simulink model "Model_120S2P"  (R2019b)
settings: Solver=VariableStepAuto  StartTime=0.0  StopTime=800  RelTol=1e-3
libraries: fl_lib x29, nesl_utility x6, simulink x2, hwlogiciolib x1, ee_lib x1
(part 2 of 3)

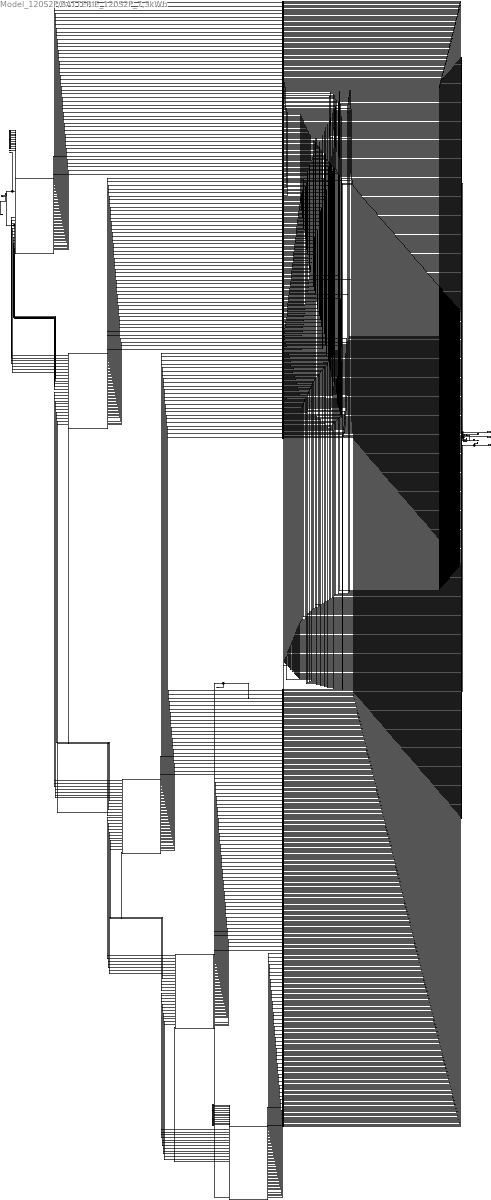
== system Model_120S2P/BATTERIE_120S2P_7,3kWh ==
  Bus Creator : BusCreator  Inputs=240
  Bus Creator1 : BusCreator  Inputs=240
  Bus Creator2 : BusCreator  Inputs=240
  Bus Selector{,1..239} (240 alike) : BusSelector  OutputSignals=Temperature,SOC,Voltage
  Compare To Constant1 : simulink/Logic and Bit Operations/Compare To Constant  relop=<=  const=0.05  OutDataTypeStr=boolean
  Compare To Constant2 : simulink/Logic and Bit Operations/Compare To Constant  relop=>  const=60.5  OutDataTypeStr=boolean
  Electrical Reference : fl_lib/Electrical/Electrical Elements/Electrical Reference
  MinMax1 : MinMax
  MinMax2 : MinMax  Function=max
  OCV : Scope
  OR : Logic  Operator=OR  IconShape=distinctive  AllPortsSameDT=off  OutDataTypeStr=boolean
  PS-Simulink Converter : nesl_utility/PS-Simulink Converter  PhysicalDomain=network_engine_domain  SubClassName=ps_output  LeftPortType=input  RightPortType=output  PseudoPeriodic=off  Frequencies=[]  Unit=inherit  AffineConversion=off
  Scope : Scope
  Subsystem{,1..4} (5 alike) : Subsystem  ReferencedSubsystem=segment_24S2P
  Temperature Source{1..24} (24 alike) : fl_lib/Thermal/Thermal Sources/Temperature Source  temperature=cell_prop.T_ext K
      settings: SourceProductName=Simscape
  To Workspace : ToWorkspace  VariableName=temperature  SaveFormat=Timeseries  SampleTime=-1
  To Workspace1 : ToWorkspace  VariableName=voltage  SaveFormat=Timeseries  SampleTime=-1
  To Workspace2 : ToWorkspace  VariableName=soc  SaveFormat=Timeseries  SampleTime=-1
  Voltage Sensor : fl_lib/Electrical/Electrical Sensors/Voltage Sensor
  + : PMIOPort  Side=Left
  - : PMIOPort  Port=2  Side=Left
  LED : Outport
  TEMP : Outport  Port=2
  SOC : Outport  Port=3
  wires:
  Bus Selector197/2 -> Bus Creator2/210  "<SOC>"
  Bus Selector199/3 -> Bus Creator1/212  "<Voltage>"
  Bus Selector226/3 -> Bus Creator1/222  "<Voltage>"
  Bus Selector191/3 -> Bus Creator1/156  "<Voltage>"
  Bus Selector119/2 -> Bus Creator2/100  "<SOC>"
  Bus Selector161/2 -> Bus Creator2/181  "<SOC>"
  Bus Selector107/2 -> Bus Creator2/116  "<SOC>"
  Bus Selector139/1 -> Bus Creator/102  "<Temperature>"
  Bus Selector72/2 -> Bus Creator2/87  "<SOC>"
  Bus Selector156/3 -> Bus Creator1/168  "<Voltage>"
  Bus Selector173/3 -> Bus Creator1/190  "<Voltage>"
  Subsystem2/14 -> Bus Selector101/1
  Subsystem3/31 -> Bus Selector179/1
  Subsystem4/31 -> Bus Selector227/1
  Subsystem4/5 -> Bus Selector222/1
  Subsystem/41 -> Bus Selector32/1
  Bus Selector213/2 -> Bus Creator2/232  "<SOC>"
  Bus Selector160/2 -> Bus Creator2/180  "<SOC>"
  Subsystem/14 -> Bus Selector13/1
  Bus Selector128/1 -> Bus Creator/144  "<Temperature>"
  Subsystem/4 -> Bus Selector3/1
  Bus Selector52/3 -> Bus Creator1/61  "<Voltage>"
  Bus Selector42/1 -> Bus Creator/29  "<Temperature>"
  Bus Selector15/3 -> Bus Creator1/16  "<Voltage>"
  Bus Selector227/2 -> Bus Creator2/223  "<SOC>"
  Subsystem2/13 -> Bus Selector100/1
  Bus Selector136/2 -> Bus Creator2/128  "<SOC>"
  Bus Selector28/2 -> Bus Creator2/37  "<SOC>"
  Bus Selector15/2 -> Bus Creator2/16  "<SOC>"
  Bus Selector108/2 -> Bus Creator2/99  "<SOC>"
  Bus Selector36/1 -> Bus Creator/27  "<Temperature>"
  Subsystem/39 -> Bus Selector30/1
  Bus Selector183/3 -> Bus Creator1/150  "<Voltage>"
  Subsystem/23 -> Bus Selector22/1
  Subsystem/48 -> Bus Selector38/1
  Bus Selector105/2 -> Bus Creator2/114  "<SOC>"
  Bus Selector163/1 -> Bus Creator/148  "<Temperature>"
  Subsystem3/24 -> Bus Selector156/1
  Bus Selector195/3 -> Bus Creator1/208  "<Voltage>"
  Bus Selector55/1 -> Bus Creator/64  "<Temperature>"
  Bus Selector113/3 -> Bus Creator1/121  "<Voltage>"
  Bus Selector59/1 -> Bus Creator/68  "<Temperature>"
  Subsystem3/17 -> Bus Selector148/1
  Bus Selector70/3 -> Bus Creator1/86  "<Voltage>"
  Bus Selector73/1 -> Bus Creator/88  "<Temperature>"
  Bus Selector74/1 -> Bus Creator/89  "<Temperature>"
  Subsystem2/33 -> Bus Selector137/1
  Bus Selector231/1 -> Bus Creator/198  "<Temperature>"
  Bus Selector190/3 -> Bus Creator1/155  "<Voltage>"
  Bus Selector101/2 -> Bus Creator2/110  "<SOC>"
  Bus Selector37/1 -> Bus Creator/45  "<Temperature>"
  Bus Selector136/3 -> Bus Creator1/128  "<Voltage>"
  Bus Selector42/3 -> Bus Creator1/29  "<Voltage>"
  Subsystem2/9 -> Bus Selector142/1
  Subsystem2/42 -> Bus Selector123/1
  Bus Selector214/1 -> Bus Creator/233  "<Temperature>"
  Bus Selector238/1 -> Bus Creator/203  "<Temperature>"
  Bus Selector202/2 -> Bus Creator2/214  "<SOC>"
  Bus Selector57/1 -> Bus Creator/66  "<Temperature>"
  Bus Selector24/3 -> Bus Creator1/25  "<Voltage>"
  Bus Selector171/3 -> Bus Creator1/189  "<Voltage>"
  Bus Selector71/2 -> Bus Creator2/52  "<SOC>"
  Bus Selector206/3 -> Bus Creator1/218  "<Voltage>"
  Bus Selector55/3 -> Bus Creator1/64  "<Voltage>"
  Subsystem3/9 -> Bus Selector186/1
  Bus Selector170/2 -> Bus Creator2/171  "<SOC>"
  Bus Selector149/1 -> Bus Creator/162  "<Temperature>"
  Bus Selector176/2 -> Bus Creator2/172  "<SOC>"
  Subsystem3/1 -> Bus Selector188/1
  Bus Selector19/3 -> Bus Creator1/20  "<Voltage>"
  Bus Selector153/3 -> Bus Creator1/165  "<Voltage>"
  Bus Selector164/2 -> Bus Creator2/183  "<SOC>"
  Bus Selector153/2 -> Bus Creator2/165  "<SOC>"
  Bus Selector133/2 -> Bus Creator2/125  "<SOC>"
  Bus Selector47/2 -> Bus Creator2/34  "<SOC>"
  Bus Selector106/2 -> Bus Creator2/115  "<SOC>"
  Subsystem1/46 -> Bus Selector81/1
  Bus Selector213/3 -> Bus Creator1/232  "<Voltage>"
  Bus Selector30/1 -> Bus Creator/39  "<Temperature>"
  Bus Selector179/2 -> Bus Creator2/175  "<SOC>"
  Bus Selector150/1 -> Bus Creator/163  "<Temperature>"
  Bus Selector18/1 -> Bus Creator/19  "<Temperature>"
  Bus Selector68/3 -> Bus Creator1/84  "<Voltage>"
  Bus Selector111/1 -> Bus Creator/119  "<Temperature>"
  Bus Selector141/2 -> Bus Creator2/104  "<SOC>"
  Bus Selector45/2 -> Bus Creator2/32  "<SOC>"
  Subsystem1/28 -> Bus Selector84/1
  Bus Selector77/2 -> Bus Creator2/92  "<SOC>"
  Subsystem1/22 -> Bus Selector62/1
  Bus Selector34/3 -> Bus Creator1/43  "<Voltage>"
  Subsystem4/47 -> Bus Selector223/1
  Subsystem3/38 -> Bus Selector162/1
  Bus Selector157/2 -> Bus Creator2/169  "<SOC>"
  Bus Selector199/2 -> Bus Creator2/212  "<SOC>"
  Subsystem1/45 -> Bus Selector79/1
  Bus Selector39/2 -> Bus Creator2/46  "<SOC>"
  Bus Selector7/2 -> Bus Creator2/8  "<SOC>"
  Subsystem4/15 -> Bus Selector194/1
  Bus Selector161/3 -> Bus Creator1/181  "<Voltage>"
  Bus Selector119/3 -> Bus Creator1/100  "<Voltage>"
  Bus Selector182/1 -> Bus Creator/178  "<Temperature>"
  Bus Selector4/2 -> Bus Creator2/5  "<SOC>"
  Bus Selector75/2 -> Bus Creator2/90  "<SOC>"
  Bus Selector113/1 -> Bus Creator/121  "<Temperature>"
  Bus Selector57/2 -> Bus Creator2/66  "<SOC>"
  Bus Selector44/2 -> Bus Creator2/31  "<SOC>"
  Bus Selector109/2 -> Bus Creator2/117  "<SOC>"
  Bus Selector120/2 -> Bus Creator2/135  "<SOC>"
  Bus Selector137/3 -> Bus Creator1/129  "<Voltage>"
  Bus Selector143/2 -> Bus Creator2/106  "<SOC>"
  Subsystem4/28 -> Bus Selector224/1
  Subsystem/38 -> Bus Selector29/1
  Bus Selector235/3 -> Bus Creator1/202  "<Voltage>"
  Bus Selector218/2 -> Bus Creator2/219  "<SOC>"
  Bus Selector200/1 -> Bus Creator/195  "<Temperature>"
  Bus Selector165/1 -> Bus Creator/184  "<Temperature>"
  Bus Selector134/1 -> Bus Creator/126  "<Temperature>"
  Bus Selector117/3 -> Bus Creator1/133  "<Voltage>"
  Subsystem2/1 -> Bus Selector96/1
  Bus Selector102/3 -> Bus Creator1/111  "<Voltage>"
  Bus Selector134/3 -> Bus Creator1/126  "<Voltage>"
  Bus Selector217/3 -> Bus Creator1/236  "<Voltage>"
  Bus Selector223/3 -> Bus Creator1/239  "<Voltage>"
  Bus Selector130/3 -> Bus Creator1/101  "<Voltage>"
  Bus Selector227/3 -> Bus Creator1/223  "<Voltage>"
  Bus Selector31/3 -> Bus Creator1/40  "<Voltage>"
  Bus Selector212/3 -> Bus Creator1/231  "<Voltage>"
  Bus Selector222/1 -> Bus Creator/197  "<Temperature>"
  Bus Selector223/1 -> Bus Creator/239  "<Temperature>"
  Bus Selector43/1 -> Bus Creator/30  "<Temperature>"
  Bus Selector78/2 -> Bus Creator2/75  "<SOC>"
  Bus Selector191/2 -> Bus Creator2/156  "<SOC>"
  Bus Selector177/3 -> Bus Creator1/173  "<Voltage>"
  Subsystem/6 -> Bus Selector5/1
  Bus Selector112/2 -> Bus Creator2/120  "<SOC>"
  Bus Selector22/2 -> Bus Creator2/23  "<SOC>"
  Subsystem/10 -> Bus Selector9/1
  Subsystem2/5 -> Bus Selector130/1
  Bus Selector90/3 -> Bus Creator1/82  "<Voltage>"
  Bus Selector140/1 -> Bus Creator/103  "<Temperature>"
  Bus Selector89/1 -> Bus Creator/81  "<Temperature>"
  Bus Selector180/3 -> Bus Creator1/176  "<Voltage>"
  Bus Selector117/2 -> Bus Creator2/133  "<SOC>"
  Bus Selector180/2 -> Bus Creator2/176  "<SOC>"
  Bus Selector45/1 -> Bus Creator/32  "<Temperature>"
  Subsystem4/29 -> Bus Selector225/1
  Bus Selector225/3 -> Bus Creator1/221  "<Voltage>"
  Bus Selector225/2 -> Bus Creator2/221  "<SOC>"
  Bus Creator1/1 -> OCV/1, To Workspace1/1
  Bus Selector64/2 -> Bus Creator2/72  "<SOC>"
  Bus Selector116/2 -> Bus Creator2/132  "<SOC>"
  Bus Selector231/2 -> Bus Creator2/198  "<SOC>"
  Bus Creator2/1 -> MinMax1/1, SOC/1, To Workspace2/1
  Subsystem3/37 -> Bus Selector161/1
  Subsystem3/8 -> Bus Selector185/1
  Subsystem1/21 -> Bus Selector61/1
  Bus Selector189/1 -> Bus Creator/146  "<Temperature>"
  Bus Selector150/3 -> Bus Creator1/163  "<Voltage>"
  Subsystem/32 -> Bus Selector45/1
  Bus Creator/1 -> MinMax2/1, TEMP/1, To Workspace/1
  Subsystem1/31 -> Bus Selector87/1
  Bus Selector9/1 -> Bus Creator/10  "<Temperature>"
  Subsystem1/27 -> Bus Selector78/1
  Bus Selector22/1 -> Bus Creator/23  "<Temperature>"
  Bus Selector154/1 -> Bus Creator/166  "<Temperature>"
  Bus Selector11/2 -> Bus Creator2/12  "<SOC>"
  Subsystem1/39 -> Bus Selector72/1
  Bus Selector60/2 -> Bus Creator2/51  "<SOC>"
  Subsystem1/36 -> Bus Selector68/1
  Bus Selector80/2 -> Bus Creator2/96  "<SOC>"
  Bus Selector12/2 -> Bus Creator2/13  "<SOC>"
  Subsystem2/26 -> Bus Selector114/1
  Subsystem3/30 -> Bus Selector178/1
  Bus Selector171/2 -> Bus Creator2/189  "<SOC>"
  Bus Selector11/3 -> Bus Creator1/12  "<Voltage>"
  Bus Selector85/3 -> Bus Creator1/77  "<Voltage>"
  Bus Selector220/3 -> Bus Creator1/240  "<Voltage>"
  Bus Selector34/2 -> Bus Creator2/43  "<SOC>"
  Bus Selector233/1 -> Bus Creator/200  "<Temperature>"
  Bus Selector184/3 -> Bus Creator1/151  "<Voltage>"
  Bus Selector82/1 -> Bus Creator/53  "<Temperature>"
  Bus Selector228/2 -> Bus Creator2/224  "<SOC>"
  Bus Selector93/2 -> Bus Creator2/56  "<SOC>"
  Subsystem4/43 -> Bus Selector216/1
  Subsystem2/15 -> Bus Selector102/1
  Bus Selector64/3 -> Bus Creator1/72  "<Voltage>"
  Bus Selector43/3 -> Bus Creator1/30  "<Voltage>"
  Bus Selector152/3 -> Bus Creator1/147  "<Voltage>"
  Subsystem4/21 -> Bus Selector201/1
  Subsystem4/27 -> Bus Selector218/1
  Bus Selector221/2 -> Bus Creator2/238  "<SOC>"
  Bus Selector145/2 -> Bus Creator2/158  "<SOC>"
  Bus Selector53/2 -> Bus Creator2/62  "<SOC>"
  Bus Selector69/2 -> Bus Creator2/85  "<SOC>"
  Subsystem1/7 -> Bus Selector92/1
  Bus Selector85/1 -> Bus Creator/77  "<Temperature>"
  Subsystem/21 -> Bus Selector20/1
  Bus Selector55/2 -> Bus Creator2/64  "<SOC>"
  Bus Selector73/3 -> Bus Creator1/88  "<Voltage>"
  Bus Selector128/2 -> Bus Creator2/144  "<SOC>"
  Bus Selector239/3 -> Bus Creator1/204  "<Voltage>"
  Bus Selector207/3 -> Bus Creator1/227  "<Voltage>"
  Bus Selector77/1 -> Bus Creator/92  "<Temperature>"
  Bus Selector62/2 -> Bus Creator2/70  "<SOC>"
  Bus Selector229/2 -> Bus Creator2/225  "<SOC>"
  Subsystem/35 -> Bus Selector26/1
  Bus Selector132/1 -> Bus Creator/124  "<Temperature>"
  Bus Selector156/1 -> Bus Creator/168  "<Temperature>"
  Subsystem1/43 -> Bus Selector76/1
  Bus Selector111/3 -> Bus Creator1/119  "<Voltage>"
  Bus Selector160/3 -> Bus Creator1/180  "<Voltage>"
  Bus Selector204/1 -> Bus Creator/216  "<Temperature>"
  Bus Selector131/2 -> Bus Creator2/143  "<SOC>"
  Bus Selector182/3 -> Bus Creator1/178  "<Voltage>"
  Subsystem/5 -> Bus Selector4/1
  Bus Selector16/2 -> Bus Creator2/17  "<SOC>"
  Bus Selector167/1 -> Bus Creator/186  "<Temperature>"
  Subsystem/15 -> Bus Selector14/1
  Subsystem4/35 -> Bus Selector207/1
  Bus Selector84/1 -> Bus Creator/76  "<Temperature>"
  Bus Selector46/2 -> Bus Creator2/33  "<SOC>"
  Subsystem3/13 -> Bus Selector144/1
  Bus Selector14/2 -> Bus Creator2/15  "<SOC>"
  Bus Selector27/2 -> Bus Creator2/36  "<SOC>"
  Bus Selector87/3 -> Bus Creator1/79  "<Voltage>"
  Subsystem4/30 -> Bus Selector226/1
  Subsystem3/28 -> Bus Selector176/1
  Subsystem1/12 -> Bus Selector51/1
  Bus Selector81/2 -> Bus Creator2/94  "<SOC>"
  Bus Selector181/2 -> Bus Creator2/177  "<SOC>"
  Bus Selector9/3 -> Bus Creator1/10  "<Voltage>"
  Bus Selector236/1 -> Bus Creator/193  "<Temperature>"
  Bus Selector226/2 -> Bus Creator2/222  "<SOC>"
  Bus Selector209/3 -> Bus Creator1/229  "<Voltage>"
  Subsystem1/2 -> Bus Selector49/1
  Bus Selector38/1 -> Bus Creator/48  "<Temperature>"
  Bus Selector154/3 -> Bus Creator1/166  "<Voltage>"
  Subsystem/24 -> Bus Selector23/1
  Subsystem3/12 -> Bus Selector191/1
  Bus Selector178/3 -> Bus Creator1/174  "<Voltage>"
  Subsystem4/2 -> Bus Selector237/1
  Bus Selector86/2 -> Bus Creator2/78  "<SOC>"
  Bus Selector208/1 -> Bus Creator/228  "<Temperature>"
  Subsystem/25 -> Bus Selector24/1
  Bus Selector105/1 -> Bus Creator/114  "<Temperature>"
  Subsystem4/17 -> Bus Selector196/1
  Bus Selector83/3 -> Bus Creator1/95  "<Voltage>"
  Bus Selector110/2 -> Bus Creator2/118  "<SOC>"
  Bus Selector210/3 -> Bus Creator1/230  "<Voltage>"
  Bus Selector13/3 -> Bus Creator1/14  "<Voltage>"
  Subsystem2/22 -> Bus Selector110/1
  Bus Selector30/2 -> Bus Creator2/39  "<SOC>"
  Bus Selector219/3 -> Bus Creator1/237  "<Voltage>"
  Bus Selector89/2 -> Bus Creator2/81  "<SOC>"
  Subsystem3/23 -> Bus Selector155/1
  Bus Selector189/2 -> Bus Creator2/146  "<SOC>"
  Subsystem4/12 -> Bus Selector239/1
  Bus Selector13/1 -> Bus Creator/14  "<Temperature>"
  Subsystem2/12 -> Bus Selector99/1
  Subsystem1/40 -> Bus Selector73/1
  Bus Selector96/2 -> Bus Creator2/97  "<SOC>"
  Bus Selector228/3 -> Bus Creator1/224  "<Voltage>"
  Bus Selector126/3 -> Bus Creator1/123  "<Voltage>"
  Bus Selector165/3 -> Bus Creator1/184  "<Voltage>"
  Bus Selector239/1 -> Bus Creator/204  "<Temperature>"
  Bus Selector89/3 -> Bus Creator1/81  "<Voltage>"
  Bus Selector52/1 -> Bus Creator/61  "<Temperature>"
  Bus Selector216/2 -> Bus Creator2/235  "<SOC>"
  Subsystem1/8 -> Bus Selector93/1
  Bus Selector148/2 -> Bus Creator2/161  "<SOC>"
  Subsystem1/33 -> Bus Selector89/1
  Subsystem1/19 -> Bus Selector58/1
  Bus Selector108/3 -> Bus Creator1/99  "<Voltage>"
  Bus Selector161/1 -> Bus Creator/181  "<Temperature>"
  Bus Selector148/1 -> Bus Creator/161  "<Temperature>"
  Bus Selector162/3 -> Bus Creator1/182  "<Voltage>"
  Bus Selector208/3 -> Bus Creator1/228  "<Voltage>"
  Subsystem1/26 -> Bus Selector66/1
  Bus Selector200/2 -> Bus Creator2/195  "<SOC>"
  Bus Selector172/3 -> Bus Creator1/192  "<Voltage>"
  Subsystem3/35 -> Bus Selector159/1
  Bus Selector203/1 -> Bus Creator/215  "<Temperature>"
  Bus Selector65/3 -> Bus Creator1/73  "<Voltage>"
  Bus Selector115/1 -> Bus Creator/131  "<Temperature>"
  Bus Selector32/1 -> Bus Creator/41  "<Temperature>"
  Compare To Constant1/1 -> OR/2
  Bus Selector86/1 -> Bus Creator/78  "<Temperature>"
  Subsystem1/30 -> Bus Selector86/1
  Bus Selector25/3 -> Bus Creator1/26  "<Voltage>"
  Subsystem/3 -> Bus Selector2/1
  Bus Selector79/2 -> Bus Creator2/93  "<SOC>"
  Bus Selector230/2 -> Bus Creator2/226  "<SOC>"
  Bus Selector194/3 -> Bus Creator1/207  "<Voltage>"
  Bus Selector181/3 -> Bus Creator1/177  "<Voltage>"
  Subsystem2/20 -> Bus Selector107/1
  Subsystem4/32 -> Bus Selector228/1
  Subsystem3/47 -> Bus Selector175/1
  Bus Selector185/1 -> Bus Creator/152  "<Temperature>"
  Bus Selector194/2 -> Bus Creator2/207  "<SOC>"
  Bus Selector6/1 -> Bus Creator/7  "<Temperature>"
  Subsystem1/5 -> Bus Selector82/1
  Bus Selector159/1 -> Bus Creator/179  "<Temperature>"
  Bus Selector78/1 -> Bus Creator/75  "<Temperature>"
  Subsystem1/3 -> Bus Selector60/1
  Bus Selector80/3 -> Bus Creator1/96  "<Voltage>"
  Bus Selector105/3 -> Bus Creator1/114  "<Voltage>"
  Bus Selector233/2 -> Bus Creator2/200  "<SOC>"
  Bus Selector76/1 -> Bus Creator/91  "<Temperature>"
  Bus Selector95/1 -> Bus Creator/58  "<Temperature>"
  Bus Selector138/2 -> Bus Creator2/130  "<SOC>"
  Bus Selector234/3 -> Bus Creator1/201  "<Voltage>"
  Subsystem1/32 -> Bus Selector88/1
  Bus Selector32/2 -> Bus Creator2/41  "<SOC>"
  Bus Selector8/2 -> Bus Creator2/9  "<SOC>"
  Bus Selector222/2 -> Bus Creator2/197  "<SOC>"
  Subsystem4/19 -> Bus Selector198/1
  Subsystem/18 -> Bus Selector17/1
  Subsystem2/35 -> Bus Selector115/1
  Bus Selector191/1 -> Bus Creator/156  "<Temperature>"
  Subsystem3/6 -> Bus Selector183/1
  Subsystem/42 -> Bus Selector33/1
  Bus Selector174/2 -> Bus Creator2/149  "<SOC>"
  Subsystem/34 -> Bus Selector47/1
  Subsystem/45 -> Bus Selector37/1
  Bus Selector56/2 -> Bus Creator2/65  "<SOC>"
  Bus Selector141/3 -> Bus Creator1/104  "<Voltage>"
  Subsystem3/32 -> Bus Selector180/1
  Bus Selector138/1 -> Bus Creator/130  "<Temperature>"
  Bus Selector100/1 -> Bus Creator/109  "<Temperature>"
  Subsystem3/36 -> Bus Selector160/1
  Bus Selector168/3 -> Bus Creator1/187  "<Voltage>"
  Bus Selector135/2 -> Bus Creator2/127  "<SOC>"
  Bus Selector44/1 -> Bus Creator/31  "<Temperature>"
  Bus Selector198/3 -> Bus Creator1/211  "<Voltage>"
  Bus Selector144/1 -> Bus Creator/157  "<Temperature>"
  Bus Selector122/2 -> Bus Creator2/137  "<SOC>"
  Subsystem2/3 -> Bus Selector108/1
  Bus Selector27/1 -> Bus Creator/36  "<Temperature>"
  Bus Selector177/1 -> Bus Creator/173  "<Temperature>"
  Subsystem2/38 -> Bus Selector118/1
  Subsystem1/35 -> Bus Selector67/1
  Bus Selector4/1 -> Bus Creator/5  "<Temperature>"
  Bus Selector43/2 -> Bus Creator2/30  "<SOC>"
  Bus Selector62/3 -> Bus Creator1/70  "<Voltage>"
  Bus Selector217/1 -> Bus Creator/236  "<Temperature>"
  Bus Selector121/1 -> Bus Creator/136  "<Temperature>"
  Bus Selector79/1 -> Bus Creator/93  "<Temperature>"
  Subsystem2/2 -> Bus Selector97/1
  Subsystem3/41 -> Bus Selector166/1
  Bus Selector39/1 -> Bus Creator/46  "<Temperature>"
  Subsystem4/4 -> Bus Selector211/1
  Bus Selector84/2 -> Bus Creator2/76  "<SOC>"
  Bus Selector184/1 -> Bus Creator/151  "<Temperature>"
  Bus Selector63/1 -> Bus Creator/71  "<Temperature>"
  Bus Selector215/3 -> Bus Creator1/234  "<Voltage>"
  Subsystem3/18 -> Bus Selector149/1
  Subsystem3/27 -> Bus Selector170/1
  Bus Selector117/1 -> Bus Creator/133  "<Temperature>"
  Bus Selector186/1 -> Bus Creator/153  "<Temperature>"
  Subsystem4/38 -> Bus Selector210/1
  Bus Selector92/3 -> Bus Creator1/55  "<Voltage>"
  Subsystem1/17 -> Bus Selector56/1
  Bus Selector21/2 -> Bus Creator2/22  "<SOC>"
  Bus Selector193/1 -> Bus Creator/206  "<Temperature>"
  Bus Selector75/3 -> Bus Creator1/90  "<Voltage>"
  Bus Selector126/1 -> Bus Creator/123  "<Temperature>"
  Bus Selector218/1 -> Bus Creator/219  "<Temperature>"
  Bus Selector143/3 -> Bus Creator1/106  "<Voltage>"
  Bus Selector71/1 -> Bus Creator/52  "<Temperature>"
  Bus Selector61/2 -> Bus Creator2/69  "<SOC>"
  Subsystem/16 -> Bus Selector15/1
  Bus Selector176/3 -> Bus Creator1/172  "<Voltage>"
  Bus Selector49/2 -> Bus Creator2/50  "<SOC>"
  Bus Selector201/2 -> Bus Creator2/213  "<SOC>"
  Bus Selector50/1 -> Bus Creator/59  "<Temperature>"
  Bus Selector170/1 -> Bus Creator/171  "<Temperature>"
  Bus Selector136/1 -> Bus Creator/128  "<Temperature>"
  Bus Selector25/2 -> Bus Creator2/26  "<SOC>"
  Bus Selector21/1 -> Bus Creator/22  "<Temperature>"
  Subsystem/40 -> Bus Selector31/1
  Bus Selector74/3 -> Bus Creator1/89  "<Voltage>"
  Bus Selector107/1 -> Bus Creator/116  "<Temperature>"
  Bus Selector54/1 -> Bus Creator/63  "<Temperature>"
  Bus Selector137/1 -> Bus Creator/129  "<Temperature>"
  Subsystem1/10 -> Bus Selector95/1
  Bus Selector193/2 -> Bus Creator2/206  "<SOC>"
  Bus Selector23/2 -> Bus Creator2/24  "<SOC>"
  Bus Selector204/2 -> Bus Creator2/216  "<SOC>"
  Bus Selector142/3 -> Bus Creator1/105  "<Voltage>"
  Bus Selector102/2 -> Bus Creator2/111  "<SOC>"
  Bus Selector174/3 -> Bus Creator1/149  "<Voltage>"
  Bus Selector236/3 -> Bus Creator1/193  "<Voltage>"
  Bus Selector37/3 -> Bus Creator1/45  "<Voltage>"
  Bus Selector110/1 -> Bus Creator/118  "<Temperature>"
  Bus Selector95/2 -> Bus Creator2/58  "<SOC>"
  Bus Selector118/1 -> Bus Creator/134  "<Temperature>"
  Bus Selector123/2 -> Bus Creator2/138  "<SOC>"
  Bus Selector212/2 -> Bus Creator2/231  "<SOC>"
  Bus Selector224/3 -> Bus Creator1/220  "<Voltage>"
  Bus Selector169/3 -> Bus Creator1/188  "<Voltage>"
  Bus Selector155/2 -> Bus Creator2/167  "<SOC>"
  Bus Selector175/1 -> Bus Creator/191  "<Temperature>"
  Bus Selector38/3 -> Bus Creator1/48  "<Voltage>"
  Subsystem2/28 -> Bus Selector132/1
  Bus Selector166/3 -> Bus Creator1/185  "<Voltage>"
  Bus Selector114/3 -> Bus Creator1/122  "<Voltage>"
  Bus Selector49/3 -> Bus Creator1/50  "<Voltage>"
  Bus Selector152/2 -> Bus Creator2/147  "<SOC>"
  Bus Selector163/3 -> Bus Creator1/148  "<Voltage>"
  Bus Selector102/1 -> Bus Creator/111  "<Temperature>"
  Bus Selector217/2 -> Bus Creator2/236  "<SOC>"
  Bus Selector118/2 -> Bus Creator2/134  "<SOC>"
  Bus Selector200/3 -> Bus Creator1/195  "<Voltage>"
  Bus Selector167/3 -> Bus Creator1/186  "<Voltage>"
  Bus Selector1/2 -> Bus Creator2/2  "<SOC>"
  Subsystem1/6 -> Bus Selector91/1
  Subsystem1/16 -> Bus Selector55/1
  Bus Selector149/2 -> Bus Creator2/162  "<SOC>"
  Subsystem3/33 -> Bus Selector181/1
  Bus Selector131/3 -> Bus Creator1/143  "<Voltage>"
  Bus Selector35/2 -> Bus Creator2/44  "<SOC>"
  Bus Selector106/1 -> Bus Creator/115  "<Temperature>"
  Bus Selector141/1 -> Bus Creator/104  "<Temperature>"
  Bus Selector3/1 -> Bus Creator/4  "<Temperature>"
  Bus Selector58/2 -> Bus Creator2/67  "<SOC>"
  Bus Selector4/3 -> Bus Creator1/5  "<Voltage>"
  Bus Selector214/3 -> Bus Creator1/233  "<Voltage>"
  Bus Selector163/2 -> Bus Creator2/148  "<SOC>"
  Bus Selector104/2 -> Bus Creator2/113  "<SOC>"
  Bus Selector210/2 -> Bus Creator2/230  "<SOC>"
  Bus Selector166/1 -> Bus Creator/185  "<Temperature>"
  Bus Selector19/1 -> Bus Creator/20  "<Temperature>"
  Bus Selector211/2 -> Bus Creator2/196  "<SOC>"
  Bus Selector229/1 -> Bus Creator/225  "<Temperature>"
  Bus Selector160/1 -> Bus Creator/180  "<Temperature>"
  Bus Selector44/3 -> Bus Creator1/31  "<Voltage>"
  Bus Selector233/3 -> Bus Creator1/200  "<Voltage>"
  Bus Selector41/3 -> Bus Creator1/28  "<Voltage>"
  Subsystem/47 -> Bus Selector40/1
  Bus Selector238/2 -> Bus Creator2/203  "<SOC>"
  Bus Selector35/3 -> Bus Creator1/44  "<Voltage>"
  Bus Selector210/1 -> Bus Creator/230  "<Temperature>"
  Subsystem4/14 -> Bus Selector193/1
  Bus Selector151/2 -> Bus Creator2/164  "<SOC>"
  Bus Selector145/1 -> Bus Creator/158  "<Temperature>"
  Bus Selector60/3 -> Bus Creator1/51  "<Voltage>"
  Subsystem3/48 -> Bus Selector172/1
  Subsystem4/44 -> Bus Selector217/1
  Bus Selector137/2 -> Bus Creator2/129  "<SOC>"
  Bus Selector237/3 -> Bus Creator1/194  "<Voltage>"
  Bus Selector34/1 -> Bus Creator/43  "<Temperature>"
  Bus Selector56/1 -> Bus Creator/65  "<Temperature>"
  Bus Selector147/3 -> Bus Creator1/160  "<Voltage>"
  Bus Selector84/3 -> Bus Creator1/76  "<Voltage>"
  Subsystem3/45 -> Bus Selector171/1
  Subsystem4/9 -> Bus Selector234/1
  Subsystem2/11 -> Bus Selector98/1
  Bus Selector53/1 -> Bus Creator/62  "<Temperature>"
  Bus Selector156/2 -> Bus Creator2/168  "<SOC>"
  Bus Selector10/3 -> Bus Creator1/11  "<Voltage>"
  Subsystem/2 -> Bus Selector1/1
  Subsystem4/37 -> Bus Selector209/1
  Bus Selector221/3 -> Bus Creator1/238  "<Voltage>"
  Bus Selector83/2 -> Bus Creator2/95  "<SOC>"
  Bus Selector65/1 -> Bus Creator/73  "<Temperature>"
  Bus Selector119/1 -> Bus Creator/100  "<Temperature>"
  Bus Selector228/1 -> Bus Creator/224  "<Temperature>"
  Bus Selector186/2 -> Bus Creator2/153  "<SOC>"
  Bus Selector232/2 -> Bus Creator2/199  "<SOC>"
  Bus Selector26/2 -> Bus Creator2/35  "<SOC>"
  Bus Selector220/2 -> Bus Creator2/240  "<SOC>"
  Subsystem4/3 -> Bus Selector200/1
  Bus Selector25/1 -> Bus Creator/26  "<Temperature>"
  Bus Selector219/2 -> Bus Creator2/237  "<SOC>"
  Bus Selector192/2 -> Bus Creator2/205  "<SOC>"
  Bus Selector138/3 -> Bus Creator1/130  "<Voltage>"
  Bus Selector131/1 -> Bus Creator/143  "<Temperature>"
  Subsystem4/33 -> Bus Selector229/1
  Bus Selector2/3 -> Bus Creator1/3  "<Voltage>"
  Subsystem/30 -> Bus Selector43/1
  Bus Selector98/3 -> Bus Creator1/107  "<Voltage>"
  Bus Selector81/1 -> Bus Creator/94  "<Temperature>"
  Bus Selector175/2 -> Bus Creator2/191  "<SOC>"
  Bus Selector173/2 -> Bus Creator2/190  "<SOC>"
  Subsystem4/6 -> Bus Selector231/1
  Bus Selector215/2 -> Bus Creator2/234  "<SOC>"
  Subsystem2/16 -> Bus Selector103/1
  Subsystem3/7 -> Bus Selector184/1
  Bus Selector197/3 -> Bus Creator1/210  "<Voltage>"
  Bus Selector12/1 -> Bus Creator/13  "<Temperature>"
  Bus Selector/2 -> Bus Creator2/1  "<SOC>"
  Bus Selector51/3 -> Bus Creator1/60  "<Voltage>"
  Subsystem4/42 -> Bus Selector215/1
  Bus Selector198/1 -> Bus Creator/211  "<Temperature>"
  Bus Selector48/2 -> Bus Creator2/49  "<SOC>"
  Subsystem2/36 -> Bus Selector116/1
  Bus Selector87/1 -> Bus Creator/79  "<Temperature>"
  Bus Selector157/1 -> Bus Creator/169  "<Temperature>"
  Subsystem4/46 -> Bus Selector221/1
  Bus Selector206/2 -> Bus Creator2/218  "<SOC>"
  Bus Selector239/2 -> Bus Creator2/204  "<SOC>"
  Bus Selector234/2 -> Bus Creator2/201  "<SOC>"
  Bus Selector155/3 -> Bus Creator1/167  "<Voltage>"
  Bus Selector76/3 -> Bus Creator1/91  "<Voltage>"
  Bus Selector135/3 -> Bus Creator1/127  "<Voltage>"
  Bus Selector166/2 -> Bus Creator2/185  "<SOC>"
  Bus Selector41/2 -> Bus Creator2/28  "<SOC>"
  Bus Selector140/3 -> Bus Creator1/103  "<Voltage>"
  Bus Selector10/1 -> Bus Creator/11  "<Temperature>"
  Subsystem3/39 -> Bus Selector164/1
  Subsystem4/20 -> Bus Selector199/1
  Bus Selector90/2 -> Bus Creator2/82  "<SOC>"
  Bus Selector75/1 -> Bus Creator/90  "<Temperature>"
  Bus Selector95/3 -> Bus Creator1/58  "<Voltage>"
  Bus Selector154/2 -> Bus Creator2/166  "<SOC>"
  Subsystem3/11 -> Bus Selector190/1
  Bus Selector100/3 -> Bus Creator1/109  "<Voltage>"
  Bus Selector125/3 -> Bus Creator1/140  "<Voltage>"
  Bus Selector27/3 -> Bus Creator1/36  "<Voltage>"
  Subsystem1/20 -> Bus Selector59/1
  Bus Selector92/2 -> Bus Creator2/55  "<SOC>"
  Subsystem3/3 -> Bus Selector152/1
  Bus Selector52/2 -> Bus Creator2/61  "<SOC>"
  Bus Selector218/3 -> Bus Creator1/219  "<Voltage>"
  Bus Selector92/1 -> Bus Creator/55  "<Temperature>"
  Bus Selector114/2 -> Bus Creator2/122  "<SOC>"
  Bus Selector169/2 -> Bus Creator2/188  "<SOC>"
  Bus Selector62/1 -> Bus Creator/70  "<Temperature>"
  Bus Selector103/2 -> Bus Creator2/112  "<SOC>"
  Subsystem2/17 -> Bus Selector104/1
  Bus Selector199/1 -> Bus Creator/212  "<Temperature>"
  Bus Selector224/2 -> Bus Creator2/220  "<SOC>"
  Bus Selector164/1 -> Bus Creator/183  "<Temperature>"
  Subsystem3/42 -> Bus Selector167/1
  Bus Selector58/1 -> Bus Creator/67  "<Temperature>"
  Bus Selector146/1 -> Bus Creator/159  "<Temperature>"
  Bus Selector224/1 -> Bus Creator/220  "<Temperature>"
  Subsystem3/4 -> Bus Selector163/1
  Bus Selector237/2 -> Bus Creator2/194  "<SOC>"
  Bus Selector35/1 -> Bus Creator/44  "<Temperature>"
  Subsystem3/40 -> Bus Selector165/1
  Subsystem4/18 -> Bus Selector197/1
  Subsystem2/10 -> Bus Selector143/1
  Bus Selector219/1 -> Bus Creator/237  "<Temperature>"
  Bus Selector88/1 -> Bus Creator/80  "<Temperature>"
  Bus Selector188/3 -> Bus Creator1/145  "<Voltage>"
  Bus Selector94/1 -> Bus Creator/57  "<Temperature>"
  Bus Selector59/3 -> Bus Creator1/68  "<Voltage>"
  Bus Selector91/2 -> Bus Creator2/54  "<SOC>"
  Bus Selector164/3 -> Bus Creator1/183  "<Voltage>"
  Bus Selector231/3 -> Bus Creator1/198  "<Voltage>"
  Subsystem2/27 -> Bus Selector126/1
  Bus Selector54/3 -> Bus Creator1/63  "<Voltage>"
  Subsystem3/43 -> Bus Selector168/1
  Subsystem2/25 -> Bus Selector113/1
  Bus Selector51/1 -> Bus Creator/60  "<Temperature>"
  Bus Selector203/3 -> Bus Creator1/215  "<Voltage>"
  Bus Selector158/2 -> Bus Creator2/170  "<SOC>"
  Bus Selector18/2 -> Bus Creator2/19  "<SOC>"
  Bus Selector213/1 -> Bus Creator/232  "<Temperature>"
  Bus Selector94/2 -> Bus Creator2/57  "<SOC>"
  Bus Selector6/2 -> Bus Creator2/7  "<SOC>"
  Bus Selector206/1 -> Bus Creator/218  "<Temperature>"
  Bus Selector76/2 -> Bus Creator2/91  "<SOC>"
  Bus Selector68/2 -> Bus Creator2/84  "<SOC>"
  Bus Selector207/2 -> Bus Creator2/227  "<SOC>"
  Bus Selector101/1 -> Bus Creator/110  "<Temperature>"
  Bus Selector11/1 -> Bus Creator/12  "<Temperature>"
  Subsystem1/29 -> Bus Selector85/1
  Bus Selector59/2 -> Bus Creator2/68  "<SOC>"
  Subsystem2/4 -> Bus Selector119/1
  Subsystem3/2 -> Bus Selector189/1
  Bus Selector97/2 -> Bus Creator2/98  "<SOC>"
  Bus Selector124/3 -> Bus Creator1/139  "<Voltage>"
  Subsystem1/4 -> Bus Selector71/1
  Bus Selector139/2 -> Bus Creator2/102  "<SOC>"
  Bus Selector57/3 -> Bus Creator1/66  "<Voltage>"
  Bus Selector146/2 -> Bus Creator2/159  "<SOC>"
  Bus Selector99/2 -> Bus Creator2/108  "<SOC>"
  Subsystem2/6 -> Bus Selector139/1
  Bus Selector168/2 -> Bus Creator2/187  "<SOC>"
  Bus Selector20/3 -> Bus Creator1/21  "<Voltage>"
  Bus Selector205/2 -> Bus Creator2/217  "<SOC>"
  Bus Selector50/2 -> Bus Creator2/59  "<SOC>"
  Bus Selector207/1 -> Bus Creator/227  "<Temperature>"
  Bus Selector211/1 -> Bus Creator/196  "<Temperature>"
  Bus Selector122/1 -> Bus Creator/137  "<Temperature>"
  Bus Selector178/1 -> Bus Creator/174  "<Temperature>"
  Bus Selector212/1 -> Bus Creator/231  "<Temperature>"
  Bus Selector235/1 -> Bus Creator/202  "<Temperature>"
  MinMax2/1 -> Compare To Constant2/1
  Bus Selector96/3 -> Bus Creator1/97  "<Voltage>"
  Subsystem3/25 -> Bus Selector157/1
  Bus Selector183/2 -> Bus Creator2/150  "<SOC>"
  Subsystem/7 -> Bus Selector6/1
  Bus Selector142/2 -> Bus Creator2/105  "<SOC>"
  Bus Selector78/3 -> Bus Creator1/75  "<Voltage>"
  Bus Selector9/2 -> Bus Creator2/10  "<SOC>"
  Bus Selector101/3 -> Bus Creator1/110  "<Voltage>"
  Bus Selector32/3 -> Bus Creator1/41  "<Voltage>"
  Bus Selector36/2 -> Bus Creator2/27  "<SOC>"
  Bus Selector73/2 -> Bus Creator2/88  "<SOC>"
  Bus Selector118/3 -> Bus Creator1/134  "<Voltage>"
  Bus Selector196/2 -> Bus Creator2/209  "<SOC>"
  Bus Selector82/3 -> Bus Creator1/53  "<Voltage>"
  Subsystem1/34 -> Bus Selector90/1
  Subsystem/43 -> Bus Selector34/1
  Bus Selector16/3 -> Bus Creator1/17  "<Voltage>"
  Bus Selector126/2 -> Bus Creator2/123  "<SOC>"
  Subsystem/22 -> Bus Selector21/1
  Subsystem4/10 -> Bus Selector235/1
  Subsystem4/11 -> Bus Selector238/1
  Bus Selector202/3 -> Bus Creator1/214  "<Voltage>"
  Bus Selector195/1 -> Bus Creator/208  "<Temperature>"
  Bus Selector70/2 -> Bus Creator2/86  "<SOC>"
  Bus Selector47/1 -> Bus Creator/34  "<Temperature>"
  Bus Selector31/2 -> Bus Creator2/40  "<SOC>"
  Bus Selector24/1 -> Bus Creator/25  "<Temperature>"
  Bus Selector174/1 -> Bus Creator/149  "<Temperature>"
  Subsystem/12 -> Bus Selector11/1
  Bus Selector63/3 -> Bus Creator1/71  "<Voltage>"
  Bus Selector29/2 -> Bus Creator2/38  "<SOC>"
  Bus Selector47/3 -> Bus Creator1/34  "<Voltage>"
  Bus Selector180/1 -> Bus Creator/176  "<Temperature>"
  Bus Selector120/1 -> Bus Creator/135  "<Temperature>"
  Bus Selector28/1 -> Bus Creator/37  "<Temperature>"
  Bus Selector77/3 -> Bus Creator1/92  "<Voltage>"
  Bus Selector22/3 -> Bus Creator1/23  "<Voltage>"
  Bus Selector159/2 -> Bus Creator2/179  "<SOC>"
  Bus Selector17/1 -> Bus Creator/18  "<Temperature>"
  Bus Selector1/1 -> Bus Creator/2  "<Temperature>"
  Bus Selector112/1 -> Bus Creator/120  "<Temperature>"
  Bus Selector179/1 -> Bus Creator/175  "<Temperature>"
  Bus Selector70/1 -> Bus Creator/86  "<Temperature>"
  Bus Selector116/3 -> Bus Creator1/132  "<Voltage>"
  Subsystem3/19 -> Bus Selector150/1
  Bus Selector20/2 -> Bus Creator2/21  "<SOC>"
  Bus Selector40/3 -> Bus Creator1/47  "<Voltage>"
  Bus Selector39/3 -> Bus Creator1/46  "<Voltage>"
  Bus Selector162/1 -> Bus Creator/182  "<Temperature>"
  Bus Selector8/3 -> Bus Creator1/9  "<Voltage>"
  Bus Selector133/3 -> Bus Creator1/125  "<Voltage>"
  Bus Selector221/1 -> Bus Creator/238  "<Temperature>"
  Bus Selector169/1 -> Bus Creator/188  "<Temperature>"
  Bus Selector133/1 -> Bus Creator/125  "<Temperature>"
  Bus Selector146/3 -> Bus Creator1/159  "<Voltage>"
  Bus Selector121/2 -> Bus Creator2/136  "<SOC>"
  Bus Selector190/2 -> Bus Creator2/155  "<SOC>"
  Bus Selector171/1 -> Bus Creator/189  "<Temperature>"
  Bus Selector38/2 -> Bus Creator2/48  "<SOC>"
  Bus Selector40/1 -> Bus Creator/47  "<Temperature>"
  Subsystem4/45 -> Bus Selector219/1
  Bus Selector5/2 -> Bus Creator2/6  "<SOC>"
  Bus Selector88/2 -> Bus Creator2/80  "<SOC>"
  Bus Selector87/2 -> Bus Creator2/79  "<SOC>"
  Bus Selector5/3 -> Bus Creator1/6  "<Voltage>"
  Bus Selector120/3 -> Bus Creator1/135  "<Voltage>"
  Subsystem/29 -> Bus Selector42/1
  Bus Selector68/1 -> Bus Creator/84  "<Temperature>"
  Bus Selector139/3 -> Bus Creator1/102  "<Voltage>"
  Bus Selector54/2 -> Bus Creator2/63  "<SOC>"
  Bus Selector30/3 -> Bus Creator1/39  "<Voltage>"
  Bus Selector235/2 -> Bus Creator2/202  "<SOC>"
  Subsystem3/26 -> Bus Selector158/1
  Subsystem3/20 -> Bus Selector151/1
  Bus Selector74/2 -> Bus Creator2/89  "<SOC>"
  Subsystem2/29 -> Bus Selector133/1
  Bus Selector232/3 -> Bus Creator1/199  "<Voltage>"
  Bus Selector226/1 -> Bus Creator/222  "<Temperature>"
  Subsystem1/9 -> Bus Selector94/1
  Bus Selector17/2 -> Bus Creator2/18  "<SOC>"
  Bus Selector46/1 -> Bus Creator/33  "<Temperature>"
  Subsystem/1 -> Bus Selector/1
  Bus Selector201/1 -> Bus Creator/213  "<Temperature>"
  Bus Selector177/2 -> Bus Creator2/173  "<SOC>"
  Bus Selector65/2 -> Bus Creator2/73  "<SOC>"
  Bus Selector69/3 -> Bus Creator1/85  "<Voltage>"
  Bus Selector187/3 -> Bus Creator1/154  "<Voltage>"
  Bus Selector66/3 -> Bus Creator1/74  "<Voltage>"
  Subsystem1/18 -> Bus Selector57/1
  Bus Selector230/1 -> Bus Creator/226  "<Temperature>"
  Subsystem4/36 -> Bus Selector208/1
  Bus Selector63/2 -> Bus Creator2/71  "<SOC>"
  Bus Selector37/2 -> Bus Creator2/45  "<SOC>"
  Bus Selector238/3 -> Bus Creator1/203  "<Voltage>"
  Bus Selector227/1 -> Bus Creator/223  "<Temperature>"
  Bus Selector14/1 -> Bus Creator/15  "<Temperature>"
  Bus Selector48/3 -> Bus Creator1/49  "<Voltage>"
  Bus Selector51/2 -> Bus Creator2/60  "<SOC>"
  Bus Selector205/1 -> Bus Creator/217  "<Temperature>"
  Bus Selector168/1 -> Bus Creator/187  "<Temperature>"
  Bus Selector67/3 -> Bus Creator1/83  "<Voltage>"
  Bus Selector64/1 -> Bus Creator/72  "<Temperature>"
  Bus Selector17/3 -> Bus Creator1/18  "<Voltage>"
  Bus Selector128/3 -> Bus Creator1/144  "<Voltage>"
  Subsystem/28 -> Bus Selector41/1
  Bus Selector36/3 -> Bus Creator1/27  "<Voltage>"
  Bus Selector230/3 -> Bus Creator1/226  "<Voltage>"
  Bus Selector195/2 -> Bus Creator2/208  "<SOC>"
  Bus Selector201/3 -> Bus Creator1/213  "<Voltage>"
  Subsystem2/40 -> Bus Selector121/1
  Subsystem4/16 -> Bus Selector195/1
  Bus Selector203/2 -> Bus Creator2/215  "<SOC>"
  Bus Selector82/2 -> Bus Creator2/53  "<SOC>"
  Bus Selector143/1 -> Bus Creator/106  "<Temperature>"
  Bus Selector122/3 -> Bus Creator1/137  "<Voltage>"
  Subsystem2/43 -> Bus Selector124/1
  Bus Selector104/1 -> Bus Creator/113  "<Temperature>"
  Bus Selector12/3 -> Bus Creator1/13  "<Voltage>"
  Subsystem4/41 -> Bus Selector214/1
  Bus Selector97/3 -> Bus Creator1/98  "<Voltage>"
  Bus Selector182/2 -> Bus Creator2/178  "<SOC>"
  Subsystem3/29 -> Bus Selector177/1
  Bus Selector86/3 -> Bus Creator1/78  "<Voltage>"
  Bus Selector97/1 -> Bus Creator/98  "<Temperature>"
  Bus Selector173/1 -> Bus Creator/190  "<Temperature>"
  Bus Selector152/1 -> Bus Creator/147  "<Temperature>"
  Bus Selector90/1 -> Bus Creator/82  "<Temperature>"
  Bus Selector107/3 -> Bus Creator1/116  "<Voltage>"
  Bus Selector158/1 -> Bus Creator/170  "<Temperature>"
  Subsystem1/41 -> Bus Selector74/1
  Bus Selector3/2 -> Bus Creator2/4  "<SOC>"
  Bus Selector13/2 -> Bus Creator2/14  "<SOC>"
  Bus Selector151/3 -> Bus Creator1/164  "<Voltage>"
  Subsystem2/32 -> Bus Selector136/1
  Bus Selector14/3 -> Bus Creator1/15  "<Voltage>"
  Bus Selector99/3 -> Bus Creator1/108  "<Voltage>"
  Subsystem3/34 -> Bus Selector182/1
  Bus Selector198/2 -> Bus Creator2/211  "<SOC>"
  Bus Selector127/2 -> Bus Creator2/141  "<SOC>"
  Bus Selector197/1 -> Bus Creator/210  "<Temperature>"
  Bus Selector72/3 -> Bus Creator1/87  "<Voltage>"
  Bus Selector129/3 -> Bus Creator1/142  "<Voltage>"
  Subsystem4/24 -> Bus Selector204/1
  Bus Selector223/2 -> Bus Creator2/239  "<SOC>"
  Subsystem3/10 -> Bus Selector187/1
  Bus Selector91/3 -> Bus Creator1/54  "<Voltage>"
  Bus Selector158/3 -> Bus Creator1/170  "<Voltage>"
  Bus Selector1/3 -> Bus Creator1/2  "<Voltage>"
  Bus Selector79/3 -> Bus Creator1/93  "<Voltage>"
  Bus Selector93/3 -> Bus Creator1/56  "<Voltage>"
  Compare To Constant2/1 -> OR/1
  Bus Selector61/3 -> Bus Creator1/69  "<Voltage>"
  Bus Selector28/3 -> Bus Creator1/37  "<Voltage>"
  Bus Selector157/3 -> Bus Creator1/169  "<Voltage>"
  Bus Selector124/2 -> Bus Creator2/139  "<SOC>"
  Bus Selector142/1 -> Bus Creator/105  "<Temperature>"
  Bus Selector147/1 -> Bus Creator/160  "<Temperature>"
  Subsystem/13 -> Bus Selector12/1
  Bus Selector123/3 -> Bus Creator1/138  "<Voltage>"
  Bus Selector229/3 -> Bus Creator1/225  "<Voltage>"
  Subsystem2/24 -> Bus Selector112/1
  Bus Selector159/3 -> Bus Creator1/179  "<Voltage>"
  Bus Selector144/3 -> Bus Creator1/157  "<Voltage>"
  Bus Selector110/3 -> Bus Creator1/118  "<Voltage>"
  Bus Selector21/3 -> Bus Creator1/22  "<Voltage>"
  Bus Selector83/1 -> Bus Creator/95  "<Temperature>"
  Subsystem2/34 -> Bus Selector138/1
  Bus Selector150/2 -> Bus Creator2/163  "<SOC>"
  Bus Selector214/2 -> Bus Creator2/233  "<SOC>"
  Bus Selector106/3 -> Bus Creator1/115  "<Voltage>"
  Bus Selector45/3 -> Bus Creator1/32  "<Voltage>"
  Bus Selector7/3 -> Bus Creator1/8  "<Voltage>"
  Subsystem1/48 -> Bus Selector80/1
  Bus Selector53/3 -> Bus Creator1/62  "<Voltage>"
  Subsystem/20 -> Bus Selector19/1
  Bus Selector216/1 -> Bus Creator/235  "<Temperature>"
  Subsystem1/42 -> Bus Selector75/1
  Bus Selector179/3 -> Bus Creator1/175  "<Voltage>"
  Bus Selector202/1 -> Bus Creator/214  "<Temperature>"
  Subsystem3/15 -> Bus Selector146/1
  Bus Selector192/1 -> Bus Creator/205  "<Temperature>"
  Bus Selector148/3 -> Bus Creator1/161  "<Voltage>"
  Bus Selector186/3 -> Bus Creator1/153  "<Voltage>"
  Bus Selector192/3 -> Bus Creator1/205  "<Voltage>"
  Bus Selector187/2 -> Bus Creator2/154  "<SOC>"
  Bus Selector121/3 -> Bus Creator1/136  "<Voltage>"
  Bus Selector23/3 -> Bus Creator1/24  "<Voltage>"
  Bus Selector/3 -> Bus Creator1/1  "<Voltage>"
  Bus Selector94/3 -> Bus Creator1/57  "<Voltage>"
  Subsystem/17 -> Bus Selector16/1
  Bus Selector125/2 -> Bus Creator2/140  "<SOC>"
  Bus Selector/1 -> Bus Creator/1  "<Temperature>"
  Subsystem4/39 -> Bus Selector212/1
  Subsystem4/23 -> Bus Selector203/1
  Bus Selector132/2 -> Bus Creator2/124  "<SOC>"
  Bus Selector185/3 -> Bus Creator1/152  "<Voltage>"
  Bus Selector129/2 -> Bus Creator2/142  "<SOC>"
  Bus Selector6/3 -> Bus Creator1/7  "<Voltage>"
  Bus Selector18/3 -> Bus Creator1/19  "<Voltage>"
  Bus Selector185/2 -> Bus Creator2/152  "<SOC>"
  Bus Selector67/1 -> Bus Creator/83  "<Temperature>"
  Bus Selector236/2 -> Bus Creator2/193  "<SOC>"
  Bus Selector234/1 -> Bus Creator/201  "<Temperature>"
  Bus Selector50/3 -> Bus Creator1/59  "<Voltage>"
  Bus Selector69/1 -> Bus Creator/85  "<Temperature>"
  Subsystem3/14 -> Bus Selector145/1
  Bus Selector125/1 -> Bus Creator/140  "<Temperature>"
  Bus Selector194/1 -> Bus Creator/207  "<Temperature>"
  Subsystem4/22 -> Bus Selector202/1
  Bus Selector98/1 -> Bus Creator/107  "<Temperature>"
  Subsystem1/1 -> Bus Selector48/1
  Bus Selector189/3 -> Bus Creator1/146  "<Voltage>"
  Bus Selector56/3 -> Bus Creator1/65  "<Voltage>"
  Bus Selector187/1 -> Bus Creator/154  "<Temperature>"
  Bus Selector134/2 -> Bus Creator2/126  "<SOC>"
  Subsystem2/37 -> Bus Selector117/1
  Bus Selector209/2 -> Bus Creator2/229  "<SOC>"
  Bus Selector19/2 -> Bus Creator2/20  "<SOC>"
  Bus Selector46/3 -> Bus Creator1/33  "<Voltage>"
  Subsystem3/44 -> Bus Selector169/1
  Bus Selector178/2 -> Bus Creator2/174  "<SOC>"
  Bus Selector103/1 -> Bus Creator/112  "<Temperature>"
  Bus Selector67/2 -> Bus Creator2/83  "<SOC>"
  Bus Selector98/2 -> Bus Creator2/107  "<SOC>"
  Bus Selector31/1 -> Bus Creator/40  "<Temperature>"
  Bus Selector147/2 -> Bus Creator2/160  "<SOC>"
  Bus Selector71/3 -> Bus Creator1/52  "<Voltage>"
  Subsystem/8 -> Bus Selector7/1
  Bus Selector104/3 -> Bus Creator1/113  "<Voltage>"
  Bus Selector153/1 -> Bus Creator/165  "<Temperature>"
  Bus Selector99/1 -> Bus Creator/108  "<Temperature>"
  Bus Selector155/1 -> Bus Creator/167  "<Temperature>"
  Bus Selector26/1 -> Bus Creator/35  "<Temperature>"
  Bus Selector190/1 -> Bus Creator/155  "<Temperature>"
  Bus Selector116/1 -> Bus Creator/132  "<Temperature>"
  Bus Selector108/1 -> Bus Creator/99  "<Temperature>"
  Bus Selector26/3 -> Bus Creator1/35  "<Voltage>"
  Subsystem2/39 -> Bus Selector120/1
  Bus Selector196/3 -> Bus Creator1/209  "<Voltage>"
  Bus Selector188/1 -> Bus Creator/145  "<Temperature>"
  Subsystem2/44 -> Bus Selector125/1
  Bus Selector151/1 -> Bus Creator/164  "<Temperature>"
  Subsystem2/47 -> Bus Selector131/1
  Bus Selector193/3 -> Bus Creator1/206  "<Voltage>"
  Bus Selector127/3 -> Bus Creator1/141  "<Voltage>"
  Bus Selector130/2 -> Bus Creator2/101  "<SOC>"
  Bus Selector33/2 -> Bus Creator2/42  "<SOC>"
  Bus Selector129/1 -> Bus Creator/142  "<Temperature>"
  Bus Selector41/1 -> Bus Creator/28  "<Temperature>"
  Bus Selector140/2 -> Bus Creator2/103  "<SOC>"
  Bus Selector127/1 -> Bus Creator/141  "<Temperature>"
  Bus Selector20/1 -> Bus Creator/21  "<Temperature>"
  Bus Selector113/2 -> Bus Creator2/121  "<SOC>"
  Bus Selector85/2 -> Bus Creator2/77  "<SOC>"
  Bus Selector130/1 -> Bus Creator/101  "<Temperature>"
  Bus Selector216/3 -> Bus Creator1/235  "<Voltage>"
  Subsystem2/31 -> Bus Selector135/1
  Bus Selector93/1 -> Bus Creator/56  "<Temperature>"
  Bus Selector208/2 -> Bus Creator2/228  "<SOC>"
  Bus Selector24/2 -> Bus Creator2/25  "<SOC>"
  Bus Selector72/1 -> Bus Creator/87  "<Temperature>"
  Subsystem4/40 -> Bus Selector213/1
  Bus Selector80/1 -> Bus Creator/96  "<Temperature>"
  Subsystem3/5 -> Bus Selector174/1
  Bus Selector144/2 -> Bus Creator2/157  "<SOC>"
  Bus Selector175/3 -> Bus Creator1/191  "<Voltage>"
  Bus Selector91/1 -> Bus Creator/54  "<Temperature>"
  Subsystem/27 -> Bus Selector36/1
  Bus Selector88/3 -> Bus Creator1/80  "<Voltage>"
  Bus Selector49/1 -> Bus Creator/50  "<Temperature>"
  Bus Selector123/1 -> Bus Creator/138  "<Temperature>"
  Bus Selector211/3 -> Bus Creator1/196  "<Voltage>"
  Bus Selector167/2 -> Bus Creator2/186  "<SOC>"
  Bus Selector181/1 -> Bus Creator/177  "<Temperature>"
  Bus Selector60/1 -> Bus Creator/51  "<Temperature>"
  Bus Selector81/3 -> Bus Creator1/94  "<Voltage>"
  Bus Selector135/1 -> Bus Creator/127  "<Temperature>"
  Bus Selector48/1 -> Bus Creator/49  "<Temperature>"
  Bus Selector10/2 -> Bus Creator2/11  "<SOC>"
  Subsystem3/21 -> Bus Selector153/1
  Bus Selector33/1 -> Bus Creator/42  "<Temperature>"
  Bus Selector109/1 -> Bus Creator/117  "<Temperature>"
  Bus Selector237/1 -> Bus Creator/194  "<Temperature>"
  Subsystem2/8 -> Bus Selector141/1
  Bus Selector170/3 -> Bus Creator1/171  "<Voltage>"
  Bus Selector205/3 -> Bus Creator1/217  "<Voltage>"
  Bus Selector29/1 -> Bus Creator/38  "<Temperature>"
  Subsystem4/8 -> Bus Selector233/1
  Subsystem2/45 -> Bus Selector127/1
  Subsystem3/16 -> Bus Selector147/1
  Bus Selector5/1 -> Bus Creator/6  "<Temperature>"
  Subsystem/36 -> Bus Selector27/1
  Bus Selector204/3 -> Bus Creator1/216  "<Voltage>"
  Bus Selector66/2 -> Bus Creator2/74  "<SOC>"
  Bus Selector96/1 -> Bus Creator/97  "<Temperature>"
  Bus Selector165/2 -> Bus Creator2/184  "<SOC>"
  Bus Selector132/3 -> Bus Creator1/124  "<Voltage>"
  Bus Selector225/1 -> Bus Creator/221  "<Temperature>"
  Bus Selector114/1 -> Bus Creator/122  "<Temperature>"
  Bus Selector8/1 -> Bus Creator/9  "<Temperature>"
  Bus Selector172/1 -> Bus Creator/192  "<Temperature>"
  Bus Selector61/1 -> Bus Creator/69  "<Temperature>"
  Bus Selector162/2 -> Bus Creator2/182  "<SOC>"
  Bus Selector3/3 -> Bus Creator1/4  "<Voltage>"
  Subsystem4/26 -> Bus Selector206/1
  Bus Selector183/1 -> Bus Creator/150  "<Temperature>"
  Subsystem4/48 -> Bus Selector220/1
  Subsystem4/34 -> Bus Selector230/1
  Subsystem1/14 -> Bus Selector53/1
  Bus Selector115/3 -> Bus Creator1/131  "<Voltage>"
  Bus Selector184/2 -> Bus Creator2/151  "<SOC>"
  Bus Selector196/1 -> Bus Creator/209  "<Temperature>"
  Subsystem4/25 -> Bus Selector205/1
  Subsystem2/7 -> Bus Selector140/1
  Bus Selector149/3 -> Bus Creator1/162  "<Voltage>"
  Bus Selector232/1 -> Bus Creator/199  "<Temperature>"
  Bus Selector112/3 -> Bus Creator1/120  "<Voltage>"
  Subsystem1/11 -> Bus Selector50/1
  Subsystem4/1 -> Bus Selector236/1
  Bus Selector58/3 -> Bus Creator1/67  "<Voltage>"
  Bus Selector29/3 -> Bus Creator1/38  "<Voltage>"
  Subsystem3/22 -> Bus Selector154/1
  Bus Selector23/1 -> Bus Creator/24  "<Temperature>"
  Subsystem/46 -> Bus Selector39/1
  Bus Selector172/2 -> Bus Creator2/192  "<SOC>"
  Bus Selector111/2 -> Bus Creator2/119  "<SOC>"
  Bus Selector2/1 -> Bus Creator/3  "<Temperature>"
  Subsystem2/19 -> Bus Selector106/1
  Subsystem/44 -> Bus Selector35/1
  Subsystem2/23 -> Bus Selector111/1
  Subsystem2/41 -> Bus Selector122/1
  Bus Selector215/1 -> Bus Creator/234  "<Temperature>"
  Bus Selector2/2 -> Bus Creator2/3  "<SOC>"
  Subsystem2/18 -> Bus Selector105/1
  Bus Selector209/1 -> Bus Creator/229  "<Temperature>"
  Bus Selector40/2 -> Bus Creator2/47  "<SOC>"
  Subsystem1/38 -> Bus Selector70/1
  Subsystem4/13 -> Bus Selector192/1
  Subsystem/11 -> Bus Selector10/1
  Subsystem4/7 -> Bus Selector232/1
  Subsystem1/15 -> Bus Selector54/1
  Subsystem/37 -> Bus Selector28/1
  Subsystem2/48 -> Bus Selector128/1
  Subsystem/33 -> Bus Selector46/1
  Bus Selector66/1 -> Bus Creator/74  "<Temperature>"
  Subsystem3/46 -> Bus Selector173/1
  Bus Selector15/1 -> Bus Creator/16  "<Temperature>"
  Subsystem/9 -> Bus Selector8/1
  Subsystem1/13 -> Bus Selector52/1
  Bus Selector188/2 -> Bus Creator2/145  "<SOC>"
  Bus Selector220/1 -> Bus Creator/240  "<Temperature>"
  Subsystem1/23 -> Bus Selector63/1
  Bus Selector124/1 -> Bus Creator/139  "<Temperature>"
  Subsystem1/37 -> Bus Selector69/1
  Subsystem/31 -> Bus Selector44/1
  Bus Selector103/3 -> Bus Creator1/112  "<Voltage>"
  Subsystem1/25 -> Bus Selector65/1
  Subsystem2/30 -> Bus Selector134/1
  Bus Selector100/2 -> Bus Creator2/109  "<SOC>"
  Bus Selector115/2 -> Bus Creator2/131  "<SOC>"
  Subsystem2/21 -> Bus Selector109/1
  Subsystem1/24 -> Bus Selector64/1
  Bus Selector7/1 -> Bus Creator/8  "<Temperature>"
  Bus Selector145/3 -> Bus Creator1/158  "<Voltage>"
  Subsystem1/44 -> Bus Selector77/1
  Bus Selector42/2 -> Bus Creator2/29  "<SOC>"
  Bus Selector222/3 -> Bus Creator1/197  "<Voltage>"
  Bus Selector33/3 -> Bus Creator1/42  "<Voltage>"
  Bus Selector109/3 -> Bus Creator1/117  "<Voltage>"
  Subsystem/26 -> Bus Selector25/1
  Bus Selector16/1 -> Bus Creator/17  "<Temperature>"
  Subsystem1/47 -> Bus Selector83/1
  Subsystem/19 -> Bus Selector18/1
  Bus Selector176/1 -> Bus Creator/172  "<Temperature>"
  Subsystem2/46 -> Bus Selector129/1
  MinMax1/1 -> Compare To Constant1/1
  OR/1 -> LED/1
  PS-Simulink Converter/1 -> Scope/1
  connections:
  Subsystem4/LConn26 -- -/RConn1 -- Electrical Reference/LConn1
  Subsystem3/LConn15 -- Subsystem4/LConn2
  Subsystem1/LConn10 -- Subsystem/LConn23
  Temperature Source4/LConn1 -- Subsystem/LConn4
  Subsystem1/LConn20 -- Subsystem2/LConn7
  Subsystem2/LConn23 -- Subsystem3/LConn10
  Subsystem/LConn24 -- Subsystem1/LConn11
  Subsystem3/LConn14 -- Subsystem4/LConn1
  Subsystem1/LConn17 -- Subsystem2/LConn4
  Subsystem1/LConn16 -- Subsystem2/LConn3
  Subsystem1/LConn26 -- Subsystem2/LConn13
  Temperature Source17/LConn1 -- Subsystem4/LConn16
  Subsystem3/LConn16 -- Subsystem4/LConn3
  Temperature Source22/LConn1 -- Subsystem4/LConn20
  Subsystem2/LConn22 -- Subsystem3/LConn9
  Subsystem1/LConn2 -- Subsystem/LConn15
  Subsystem1/LConn15 -- Subsystem2/LConn2
  Temperature Source11/LConn1 -- Subsystem/LConn11
  Subsystem2/LConn25 -- Subsystem3/LConn12
  Subsystem/LConn13 -- Voltage Sensor/LConn1 -- +/RConn1
  Temperature Source5/LConn1 -- Subsystem/LConn5
  Subsystem2/LConn20 -- Subsystem3/LConn7
  Temperature Source13/LConn1 -- Subsystem4/LConn15
  Subsystem3/LConn17 -- Subsystem4/LConn4
  Temperature Source18/LConn1 -- Subsystem4/LConn14
  Subsystem1/LConn22 -- Subsystem2/LConn9
  Subsystem3/LConn20 -- Subsystem4/LConn7
  Subsystem/LConn20 -- Subsystem1/LConn7
  Temperature Source3/LConn1 -- Subsystem/LConn1
  Temperature Source9/LConn1 -- Subsystem/LConn9
  Temperature Source8/LConn1 -- Subsystem/LConn8
  Subsystem2/LConn16 -- Subsystem3/LConn3
  Subsystem1/LConn23 -- Subsystem2/LConn10
  Subsystem/LConn17 -- Subsystem1/LConn4
  Subsystem1/LConn24 -- Subsystem2/LConn11
  Subsystem/LConn14 -- Subsystem1/LConn1
  Temperature Source1/LConn1 -- Subsystem/LConn2
  Subsystem/LConn21 -- Subsystem1/LConn8
  Subsystem2/LConn18 -- Subsystem3/LConn5
  Subsystem3/LConn21 -- Subsystem4/LConn8
  Subsystem3/LConn22 -- Subsystem4/LConn9
  Subsystem3/LConn25 -- Subsystem4/LConn12
  Subsystem2/LConn24 -- Subsystem3/LConn11
  Temperature Source7/LConn1 -- Subsystem/LConn7
  Subsystem1/LConn21 -- Subsystem2/LConn8
  Subsystem/LConn16 -- Subsystem1/LConn3
  Subsystem2/LConn14 -- Subsystem3/LConn1
  Subsystem3/LConn18 -- Subsystem4/LConn5
  Subsystem/LConn22 -- Subsystem1/LConn9
  Subsystem1/LConn25 -- Subsystem2/LConn12
  Temperature Source24/LConn1 -- Subsystem4/LConn22
  Temperature Source14/LConn1 -- Subsystem4/LConn23
  Temperature Source2/LConn1 -- Subsystem/LConn3
  Subsystem/LConn18 -- Subsystem1/LConn5
  Temperature Source20/LConn1 -- Subsystem4/LConn18
  Subsystem3/LConn24 -- Subsystem4/LConn11
  Subsystem3/LConn19 -- Subsystem4/LConn6
  Temperature Source15/LConn1 -- Subsystem4/LConn24
  Temperature Source23/LConn1 -- Subsystem4/LConn21
  Temperature Source21/LConn1 -- Subsystem4/LConn19
  Subsystem3/LConn23 -- Subsystem4/LConn10
  Subsystem2/LConn15 -- Subsystem3/LConn2
  Temperature Source10/LConn1 -- Subsystem/LConn10
  Subsystem1/LConn18 -- Subsystem2/LConn5
  Subsystem/LConn26 -- Voltage Sensor/RConn2 -- Subsystem1/LConn13
  Temperature Source16/LConn1 -- Subsystem4/LConn25
  Subsystem2/LConn26 -- Subsystem3/LConn13
  Temperature Source19/LConn1 -- Subsystem4/LConn17
  Subsystem2/LConn17 -- Subsystem3/LConn4
  Subsystem3/LConn26 -- Subsystem4/LConn13
  Subsystem1/LConn19 -- Subsystem2/LConn6
  Temperature Source6/LConn1 -- Subsystem/LConn6
  Subsystem2/LConn19 -- Subsystem3/LConn6
  Subsystem/LConn19 -- Subsystem1/LConn6
  Temperature Source12/LConn1 -- Subsystem/LConn12
  Subsystem2/LConn21 -- Subsystem3/LConn8
  Subsystem1/LConn12 -- Subsystem/LConn25
  Subsystem1/LConn14 -- Subsystem2/LConn1
  Voltage Sensor/RConn1 -- PS-Simulink Converter/LConn1
